simulink model "avang_2d_free"  (Simulink 7.8)
settings: Solver=ode45  StartTime=0.0  StopTime=10.0  RelTol=1e-3
settings Model: Creator=nike  LastModifiedBy=nike

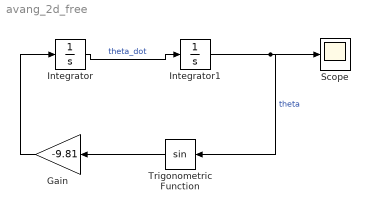
== system avang_2d_free ==
  Gain : Gain  Gain=-9.81
  Integrator : Integrator
  Integrator1 : Integrator  InitialCondition=pi/3
  Scope : Scope
  Trigonometric Function : Trigonometry
  wires:
  Integrator/1 -> Integrator1/1  "theta_dot"
  Integrator1/1 -> Trigonometric Function/1, Scope/1  "theta"
  Trigonometric Function/1 -> Gain/1
  Gain/1 -> Integrator/1
